simulink model "population_growth"  (R2022a)
settings: Solver=VariableStepAuto  StartTime=0.0  StopTime=10.0  RelTol=1e-3
settings Model: Creator=Home computer  LastModifiedBy=Home computer

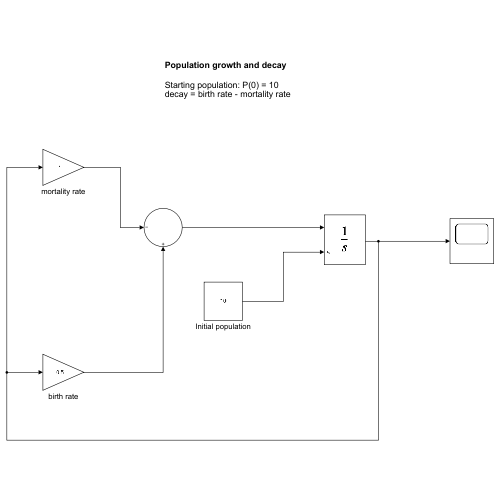
[thumbnail: Simulink's stored preview of the top-level diagram]
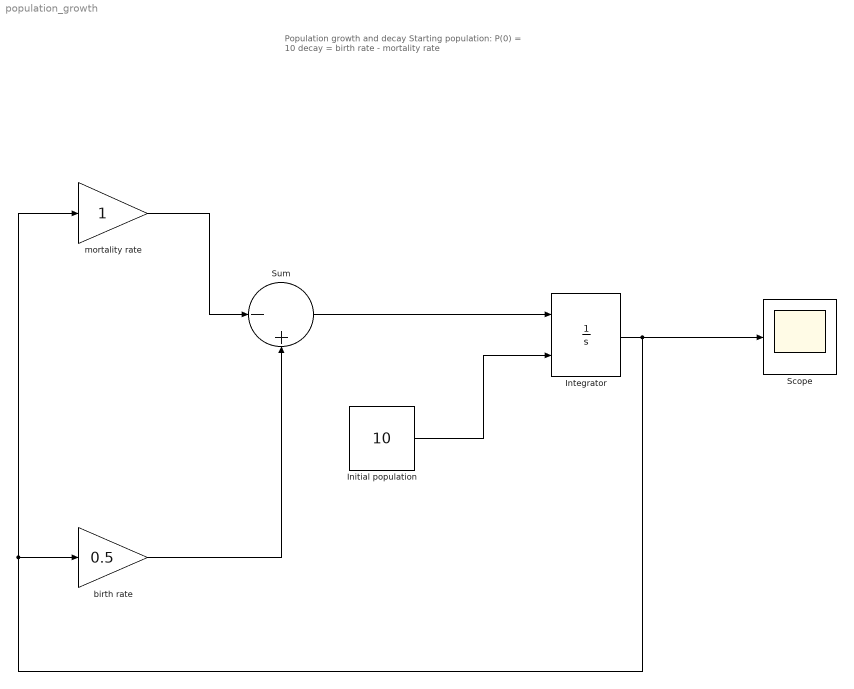
== system population_growth ==
  note: Population growth and decay
      |
      | Starting population: P(0) = 10
      | decay = birth rate - mortality rate
  Initial population : Constant  Value=10
  Integrator : Integrator  InitialConditionSource=external
  Scope : Scope
  Sum : Sum  Inputs=|-+
  birth rate : Gain  Gain=0.5
  mortality rate : Gain
  wires:
  birth rate/1 -> Sum/2
  mortality rate/1 -> Sum/1
  Sum/1 -> Integrator/1
  Integrator/1 -> Scope/1, mortality rate/1, birth rate/1
  Initial population/1 -> Integrator/2
